simulink model "Stabilization_simulink"  (R2025b)
settings: Solver=ode4  StartTime=0.0  StopTime=1  FixedStep=1/200  RelTol=1e-3
values from neighbouring files (symbols this model uses):
  dz = 28*(pi/180)    (= 0.488692190558)    [Designation_Loop_2ndTF.m]    (also in Designation_Loop_Design.m; Stabilization_Loop_Design.m)
  input_deg = 5    [Designation_Loop_2ndTF.m]    (also in Designation_Loop_Design.m; Stabilization_Loop_Design.m)
  Ki = Wc^2 / Km    (= 57.6403482438)    [Stabilization_Loop_Design.m]
  Km = 9.993    [Designation_Loop_2ndTF.m]    (also in Designation_Loop_Design.m; Performance_graph.m; Stabilization_Loop_Design.m; desig_polePlacement.m = 13.55)
  Kp = Wc^2 / Km    (= 57.6403482438)    [Designation_Loop_2ndTF.m]    (also in Designation_Loop_Design.m = 72.951065746; Performance_graph.m = Wc^2 / Km; Stabilization_Loop_Design.m = 1.79425597919; desig_polePlacement.m = 75.5719557196)
  Pm = 10.87    [Designation_Loop_2ndTF.m]    (also in Designation_Loop_Design.m; Performance_graph.m; Stabilization_Loop_Design.m; desig_polePlacement.m = 14.06)
  W_sat = 1400    [Designation_Loop_2ndTF.m]    (also in Designation_Loop_Design.m; Stabilization_Loop_Design.m)
  wb_dist = 10    [Stabilization_Loop_Design.m]
settings Model: Creator=chaeeun  LastModifiedBy=ADMIN

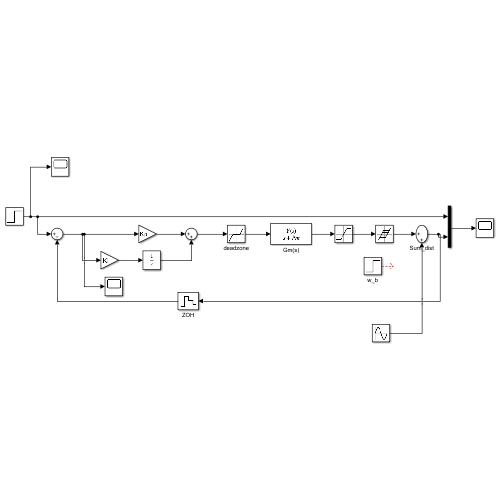
[thumbnail: Simulink's stored preview of the top-level diagram]
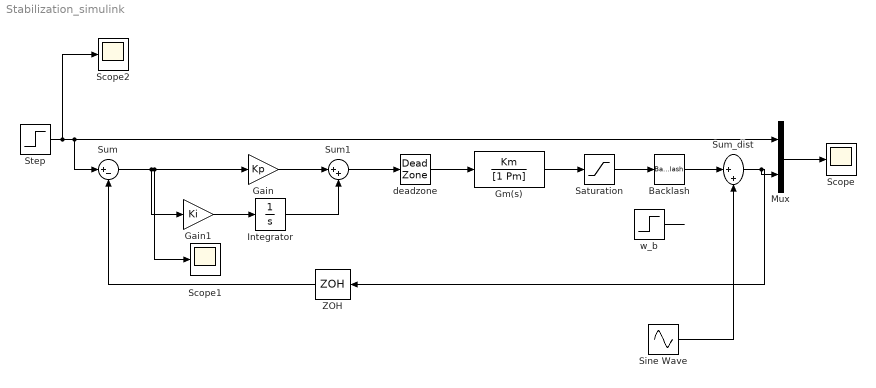
== system Stabilization_simulink ==
  Backlash : Backlash  BacklashWidth=3
  Gain : Gain  Gain=Kp
  Gain1 : Gain  Gain=Ki
  Gm(s) : TransferFcn  Numerator=Km  Denominator=[1 Pm]
  Integrator : Integrator
  Mux : Mux  Inputs=2
  Saturation : Saturate  UpperLimit=W_sat  LowerLimit=-W_sat
  Scope : Scope
      settings: ActiveDisplayYMinimum=-10.118946960587017  ActiveDisplayYMaximum=15.075027346877537
  Scope1 : Scope
      settings: ActiveDisplayYMinimum=-1  ActiveDisplayYMaximum=1
  Scope2 : Scope
      settings: ActiveDisplayYMinimum=-1  ActiveDisplayYMaximum=1  DataLoggingVariableName=ScopeData2
  Sine Wave : Sin  Frequency=0.5*2*pi  SampleTime=0
  Step : Step  Time=0  After=input_deg  SampleTime=0  VectorParams1D=off
  Sum : Sum  Inputs=|+-
  Sum1 : Sum  Inputs=|++
  Sum_dist : Sum  Inputs=|++
  ZOH : ZeroOrderHold  SampleTime=1/200
  deadzone : DeadZone  LowerValue=-dz  UpperValue=dz
  w_b : Step  Time=0.25  After=wb_dist  SampleTime=0  VectorParams1D=off
  wires:
  ZOH/1 -> Sum/2
  Mux/1 -> Scope/1
  Sum_dist/1 -> ZOH/1, Mux/2
  Step/1 -> Scope2/1, Mux/1, Sum/1
  Gain/1 -> Sum1/1
  Sum/1 -> Gain/1, Scope1/1, Gain1/1
  Gain1/1 -> Integrator/1
  Integrator/1 -> Sum1/2
  Sum1/1 -> deadzone/1
  deadzone/1 -> Gm(s)/1
  Gm(s)/1 -> Saturation/1
  Saturation/1 -> Backlash/1
  Backlash/1 -> Sum_dist/1
  w_b/1 -> ?
  Sine Wave/1 -> Sum_dist/2
